simulink model "TRN_V3"  (R2022a)
settings: Solver=FixedStepAuto  StartTime=0.0  StopTime=300  FixedStep=0.04  RelTol=1e-3
PreLoadFcn:
  | load('BusStructureTRNsensor.mat')
InitFcn:
  | %load TRNDataBusPILS.mat
  | %addpath(genpath(cd))
  | 
  | % Add DataBus Path
  | addpath(',,/');
  | addpath('../MAP/');
  | addpath('../MAP/MAP_DB');
  | addpath('../MAP/DVOF');
  | addpath(genpath(cd));
  | load('BusStructureTRN.mat');
  | load('BusStructureDatapump.mat');
undefined symbols (not defined in the file or in its folder): Altitude_INS, INSDataNotValid, Latitude_INS, Longitude_INS, RALTValid, TRN, TRNlib
libraries: simulink_extras x38, aerolibconvert2 x20, dspstat3 x3, sharedtransform x2
(part 2 of 3)

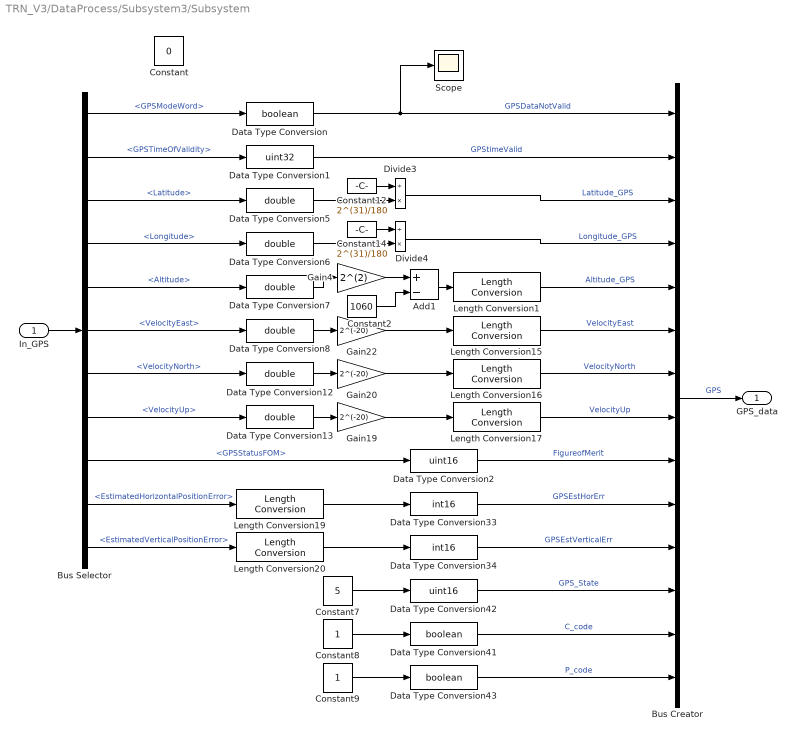
== system TRN_V3/DataProcess/Subsystem3/Subsystem ==
  In_GPS : Inport
  Add1 : Sum  Inputs=+-
  Bus Creator : BusCreator  Inputs=14  OutDataTypeStr=Bus: TRN_GPS
  Bus Selector : BusSelector  OutputSignals=GPSModeWord,GPSTimeOfValidity,Latitude,Longitude,Altitude,VelocityEast,VelocityNorth,VelocityUp,GPSStatusFOM,EstimatedHorizontalPositionError,EstimatedVerticalPositionError
  Constant : Constant  Value=0
  Constant12 : Constant  Value=2^(31)/180
  Constant14 : Constant  Value=2^(31)/180
  Constant2 : Constant  Value=1060
  Constant7 : Constant  Value=5
  Constant8 : Constant
  Constant9 : Constant
  Data Type Conversion : DataTypeConversion  OutDataTypeStr=boolean  SaturateOnIntegerOverflow=off  RndMeth=Floor
  Data Type Conversion1 : DataTypeConversion  OutDataTypeStr=uint32  SaturateOnIntegerOverflow=off  RndMeth=Floor
  Data Type Conversion{5..8,12..13} (6 alike) : DataTypeConversion  OutDataTypeStr=double  SaturateOnIntegerOverflow=off  RndMeth=Floor
  Data Type Conversion2 : DataTypeConversion  OutDataTypeStr=uint16  SaturateOnIntegerOverflow=off  RndMeth=Floor
  Data Type Conversion33 : DataTypeConversion  OutDataTypeStr=int16  SaturateOnIntegerOverflow=off  RndMeth=Floor
  Data Type Conversion34 : DataTypeConversion  OutDataTypeStr=int16  SaturateOnIntegerOverflow=off  RndMeth=Floor
  Data Type Conversion41 : DataTypeConversion  OutDataTypeStr=boolean  SaturateOnIntegerOverflow=off  RndMeth=Floor
  Data Type Conversion42 : DataTypeConversion  OutDataTypeStr=uint16  SaturateOnIntegerOverflow=off  RndMeth=Floor
  Data Type Conversion43 : DataTypeConversion  OutDataTypeStr=boolean  SaturateOnIntegerOverflow=off  RndMeth=Floor
  Divide3 : Product  Inputs=/*
  Divide4 : Product  Inputs=/*
  Gain19 : Gain  Gain=2^(-20)
  Gain20 : Gain  Gain=2^(-20)
  Gain22 : Gain  Gain=2^(-20)
  Gain4 : Gain  Gain=2^(2)
  Length Conversion{1,15..17,19..20} (6 alike) : aerolibconvert2/Length Conversion  IU=ft  OU=m
  Scope : Scope
  GPS_data : Outport
  wires:
  Length Conversion1/1 -> Bus Creator/5  "Altitude_GPS"
  Bus Selector/7 -> Data Type Conversion12/1  "<VelocityNorth>"
  Bus Selector/2 -> Data Type Conversion1/1  "<GPSTimeOfValidity>"
  Bus Selector/3 -> Data Type Conversion5/1  "<Latitude>"
  Gain4/1 -> Add1/1
  Data Type Conversion33/1 -> Bus Creator/10  "GPSEstHorErr"
  Bus Selector/5 -> Data Type Conversion7/1  "<Altitude>"
  Data Type Conversion8/1 -> Gain22/1
  Data Type Conversion41/1 -> Bus Creator/13  "C_code"
  Bus Selector/11 -> Length Conversion20/1  "<EstimatedVerticalPositionError>"
  Gain20/1 -> Length Conversion16/1
  Bus Selector/10 -> Length Conversion19/1  "<EstimatedHorizontalPositionError>"
  Divide3/1 -> Bus Creator/3  "Latitude_GPS"
  Bus Selector/6 -> Data Type Conversion8/1  "<VelocityEast>"
  Data Type Conversion13/1 -> Gain19/1
  Data Type Conversion6/1 -> Divide4/2
  Data Type Conversion34/1 -> Bus Creator/11  "GPSEstVerticalErr"
  Data Type Conversion42/1 -> Bus Creator/12  "GPS_State"
  Gain22/1 -> Length Conversion15/1
  Length Conversion20/1 -> Data Type Conversion34/1
  Data Type Conversion5/1 -> Divide3/2
  Add1/1 -> Length Conversion1/1
  Data Type Conversion1/1 -> Bus Creator/2  "GPStimeValid"
  Gain19/1 -> Length Conversion17/1
  Constant8/1 -> Data Type Conversion41/1
  Data Type Conversion2/1 -> Bus Creator/9  "FigureofMerit"
  Data Type Conversion7/1 -> Gain4/1
  Bus Selector/8 -> Data Type Conversion13/1  "<VelocityUp>"
  Constant7/1 -> Data Type Conversion42/1
  Bus Selector/4 -> Data Type Conversion6/1  "<Longitude>"
  Bus Selector/9 -> Data Type Conversion2/1  "<GPSStatusFOM>"
  Length Conversion17/1 -> Bus Creator/8  "VelocityUp"
  Length Conversion16/1 -> Bus Creator/7  "VelocityNorth"
  Bus Creator/1 -> GPS_data/1  "GPS"
  Data Type Conversion12/1 -> Gain20/1
  Constant2/1 -> Add1/2
  Length Conversion15/1 -> Bus Creator/6  "VelocityEast"
  Length Conversion19/1 -> Data Type Conversion33/1
  Divide4/1 -> Bus Creator/4  "Longitude_GPS"
  Constant9/1 -> Data Type Conversion43/1
  In_GPS/1 -> Bus Selector/1
  Constant14/1 -> Divide4/1
  Constant12/1 -> Divide3/1
  Data Type Conversion43/1 -> Bus Creator/14  "P_code"
  Data Type Conversion/1 -> Scope/1, Bus Creator/1  "GPSDataNotValid"
  Bus Selector/1 -> Data Type Conversion/1  "<GPSModeWord>"

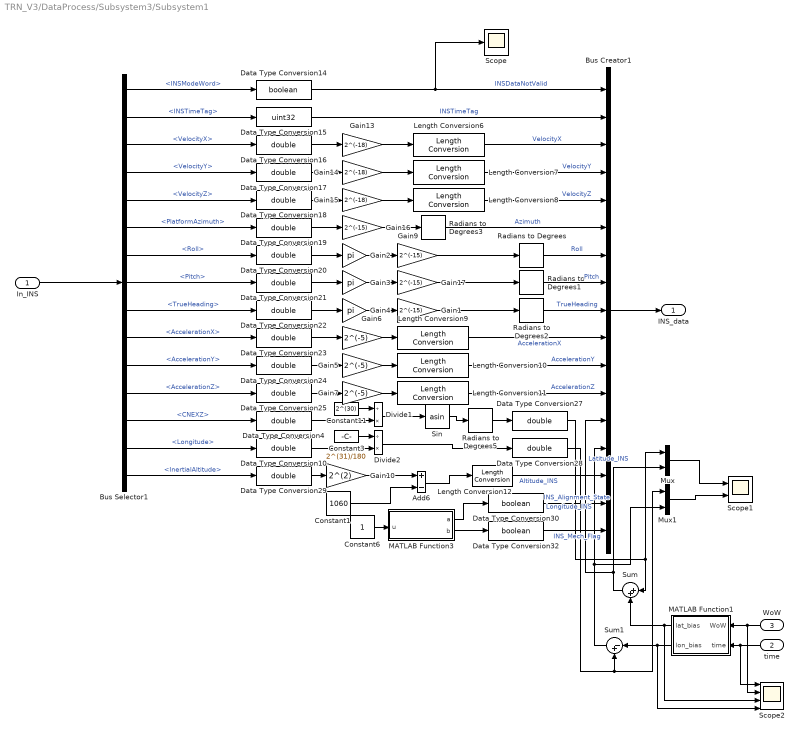
== system TRN_V3/DataProcess/Subsystem3/Subsystem1 ==
  In_INS : Inport
  time : Inport  Port=2
  WoW : Inport  Port=3
  Add6 : Sum  Inputs=+-
  Bus Creator1 : BusCreator  Inputs=17  OutDataTypeStr=Bus: TRN_INS
  Bus Selector1 : BusSelector  OutputSignals=INSModeWord,INSTimeTag,VelocityX,VelocityY,VelocityZ,PlatformAzimuth,Roll,Pitch,TrueHeading,AccelerationX,AccelerationY,AccelerationZ,CNEXZ,Longitude,InertialAltitude
  Constant1 : Constant  Value=1060
  Constant11 : Constant  Value=2^(30)
  Constant3 : Constant  Value=2^(31)/180
  Constant6 : Constant
  Data Type Conversion{4,10,16..25,27..29} (15 alike) : DataTypeConversion  OutDataTypeStr=double  SaturateOnIntegerOverflow=off  RndMeth=Floor
  Data Type Conversion14 : DataTypeConversion  OutDataTypeStr=boolean  SaturateOnIntegerOverflow=off  RndMeth=Floor
  Data Type Conversion15 : DataTypeConversion  OutDataTypeStr=uint32  SaturateOnIntegerOverflow=off  RndMeth=Floor
  Data Type Conversion30 : DataTypeConversion  OutDataTypeStr=boolean  SaturateOnIntegerOverflow=off  RndMeth=Floor
  Data Type Conversion32 : DataTypeConversion  OutDataTypeStr=boolean  SaturateOnIntegerOverflow=off  RndMeth=Floor
  Divide1 : Product  Inputs=/*
  Divide2 : Product  Inputs=/*
  Gain{1,9,16..17} (4 alike) : Gain  Gain=2^(-15)
  Gain10 : Gain  Gain=2^(2)
  Gain13 : Gain  Gain=2^(-18)
  Gain14 : Gain  Gain=2^(-18)
  Gain15 : Gain  Gain=2^(-18)
  Gain2 : Gain  Gain=pi
  Gain3 : Gain  Gain=pi
  Gain4 : Gain  Gain=pi
  Gain5 : Gain  Gain=2^(-5)
  Gain6 : Gain  Gain=2^(-5)
  Gain7 : Gain  Gain=2^(-5)
  Length Conversion{6..12} (7 alike) : aerolibconvert2/Length Conversion  IU=ft  OU=m
  MATLAB Function1 : MATLAB Function  TreatAsAtomicUnit=on
  MATLAB Function3 : MATLAB Function  TreatAsAtomicUnit=on
  Mux : Mux  Inputs=2
  Mux1 : Mux  Inputs=2
  Radians to Degrees{,1..3,5} (5 alike) : simulink_extras/Transformations/Radians to Degrees
  Scope : Scope
  Scope1 : Scope  NumInputPorts=2
  Scope2 : Scope  NumInputPorts=4
  Sin : Trigonometry  Operator=asin
  Sum : Sum  Inputs=|++
  Sum1 : Sum  Inputs=|-+
  INS_data : Outport
  wires:
  Length Conversion6/1 -> Bus Creator1/3  "VelocityX"
  Constant6/1 -> MATLAB Function3/1(u)
  MATLAB Function3/2(b) -> Data Type Conversion32/1
  Data Type Conversion32/1 -> Bus Creator1/17  "INS_Mech_Flag"
  Data Type Conversion22/1 -> Gain4/1
  Length Conversion9/1 -> Bus Creator1/10  "AccelerationX"
  Data Type Conversion29/1 -> Gain10/1
  Radians to Degrees2/1 -> Bus Creator1/9  "TrueHeading"
  Data Type Conversion16/1 -> Gain13/1
  Data Type Conversion18/1 -> Gain15/1
  Data Type Conversion15/1 -> Bus Creator1/2  "INSTimeTag"
  Bus Selector1/14 -> Data Type Conversion10/1  "<Longitude>"
  Radians to Degrees5/1 -> Data Type Conversion27/1
  Data Type Conversion24/1 -> Gain5/1
  Sin/1 -> Radians to Degrees5/1
  Constant1/1 -> Add6/2
  Gain14/1 -> Length Conversion7/1
  Data Type Conversion14/1 -> Scope/1, Bus Creator1/1  "INSDataNotValid"
  Bus Selector1/5 -> Data Type Conversion18/1  "<VelocityZ>"
  Data Type Conversion25/1 -> Gain7/1
  Divide2/1 -> Data Type Conversion28/1
  MATLAB Function3/1(a) -> Data Type Conversion30/1
  Data Type Conversion19/1 -> Gain16/1
  Bus Selector1/10 -> Data Type Conversion23/1  "<AccelerationX>"
  Data Type Conversion20/1 -> Gain2/1
  Bus Selector1/6 -> Data Type Conversion19/1  "<PlatformAzimuth>"
  Data Type Conversion23/1 -> Gain6/1
  Bus Selector1/7 -> Data Type Conversion20/1  "<Roll>"
  Bus Selector1/2 -> Data Type Conversion15/1  "<INSTimeTag>"
  Bus Selector1/4 -> Data Type Conversion17/1  "<VelocityY>"
  Bus Selector1/3 -> Data Type Conversion16/1  "<VelocityX>"
  Add6/1 -> Length Conversion12/1
  Bus Selector1/15 -> Data Type Conversion29/1  "<InertialAltitude>"
  Bus Selector1/12 -> Data Type Conversion25/1  "<AccelerationZ>"
  Bus Selector1/13 -> Data Type Conversion4/1  "<CNEXZ>"
  Data Type Conversion4/1 -> Divide1/2
  Bus Selector1/9 -> Data Type Conversion22/1  "<TrueHeading>"
  Gain15/1 -> Length Conversion8/1
  Bus Selector1/11 -> Data Type Conversion24/1  "<AccelerationY>"
  Length Conversion12/1 -> Bus Creator1/15  "Altitude_INS"
  Gain6/1 -> Length Conversion9/1
  Data Type Conversion21/1 -> Gain3/1
  Length Conversion8/1 -> Bus Creator1/5  "VelocityZ"
  Data Type Conversion17/1 -> Gain14/1
  Radians to Degrees1/1 -> Bus Creator1/8  "Pitch"
  Length Conversion7/1 -> Bus Creator1/4  "VelocityY"
  Constant3/1 -> Divide2/1
  Gain5/1 -> Length Conversion10/1
  Length Conversion10/1 -> Bus Creator1/11  "AccelerationY"
  Gain7/1 -> Length Conversion11/1
  Radians to Degrees/1 -> Bus Creator1/7  "Roll"
  Divide1/1 -> Sin/1
  Bus Selector1/8 -> Data Type Conversion21/1  "<Pitch>"
  Data Type Conversion10/1 -> Divide2/2
  Data Type Conversion30/1 -> Bus Creator1/16  "INS_Alignment_State"
  Gain10/1 -> Add6/1
  Radians to Degrees3/1 -> Bus Creator1/6  "Azimuth"
  Length Conversion11/1 -> Bus Creator1/12  "AccelerationZ"
  Constant11/1 -> Divide1/1
  Gain16/1 -> Radians to Degrees3/1
  Gain13/1 -> Length Conversion6/1
  Bus Creator1/1 -> INS_data/1
  In_INS/1 -> Bus Selector1/1
  Gain3/1 -> Gain17/1
  Gain4/1 -> Gain1/1
  Gain2/1 -> Gain9/1
  Gain9/1 -> Radians to Degrees/1
  Gain17/1 -> Radians to Degrees1/1
  Gain1/1 -> Radians to Degrees2/1
  Bus Selector1/1 -> Data Type Conversion14/1  "<INSModeWord>"
  Sum/1 -> Bus Creator1/13, Mux/2  "Latitude_INS"
  MATLAB Function1/1(lat_bias) -> Scope2/3, Sum/2
  Sum1/1 -> Mux1/2, Bus Creator1/14  "Longitude_INS"
  MATLAB Function1/2(lon_bias) -> Scope2/4, Sum1/1
  Mux/1 -> Scope1/1
  Mux1/1 -> Scope1/2
  Data Type Conversion27/1 -> Sum/1, Mux/1
  Data Type Conversion28/1 -> Sum1/2, Mux1/1
  WoW/1 -> Scope2/2, MATLAB Function1/1(WoW)
  time/1 -> Scope2/1, MATLAB Function1/2(time)

== system TRN_V3/DataProcess/Subsystem3/Subsystem4 ==
  In_RALT : Inport
  Add5 : Sum  Inputs=+-
  Bus Creator2 : BusCreator  Inputs=3  OutDataTypeStr=Bus: TRN_RALT
  Bus Selector2 : BusSelector  OutputSignals=RALTModeWord,TimeTag,RadarAltitude
  Constant4 : Constant  Value=50
  Constant5 : Constant  Value=0.625
  Data Type Conversion3 : DataTypeConversion  OutDataTypeStr=double  SaturateOnIntegerOverflow=off  RndMeth=Floor
  Data Type Conversion31 : DataTypeConversion  OutDataTypeStr=uint32  SaturateOnIntegerOverflow=off  RndMeth=Floor
  Data Type Conversion35 : DataTypeConversion  OutDataTypeStr=boolean  SaturateOnIntegerOverflow=off  RndMeth=Floor
  Length Conversion2 : aerolibconvert2/Length Conversion  IU=ft  OU=m
  Product1 : Product
  RALT_data : Outport
  wires:
  Length Conversion2/1 -> Bus Creator2/3  "RALTAltitude"
  Constant4/1 -> Add5/2
  Bus Creator2/1 -> RALT_data/1  "RALT"
  In_RALT/1 -> Bus Selector2/1
  Data Type Conversion35/1 -> Bus Creator2/1  "RALTValid"
  Add5/1 -> Length Conversion2/1
  Bus Selector2/3 -> Data Type Conversion3/1  "<RadarAltitude>"
  Data Type Conversion3/1 -> Product1/1
  Product1/1 -> Add5/1
  Constant5/1 -> Product1/2
  Data Type Conversion31/1 -> Bus Creator2/2  "RALTTimeTag"
  Bus Selector2/2 -> Data Type Conversion31/1  "<TimeTag>"
  Bus Selector2/1 -> Data Type Conversion35/1  "<RALTModeWord>"

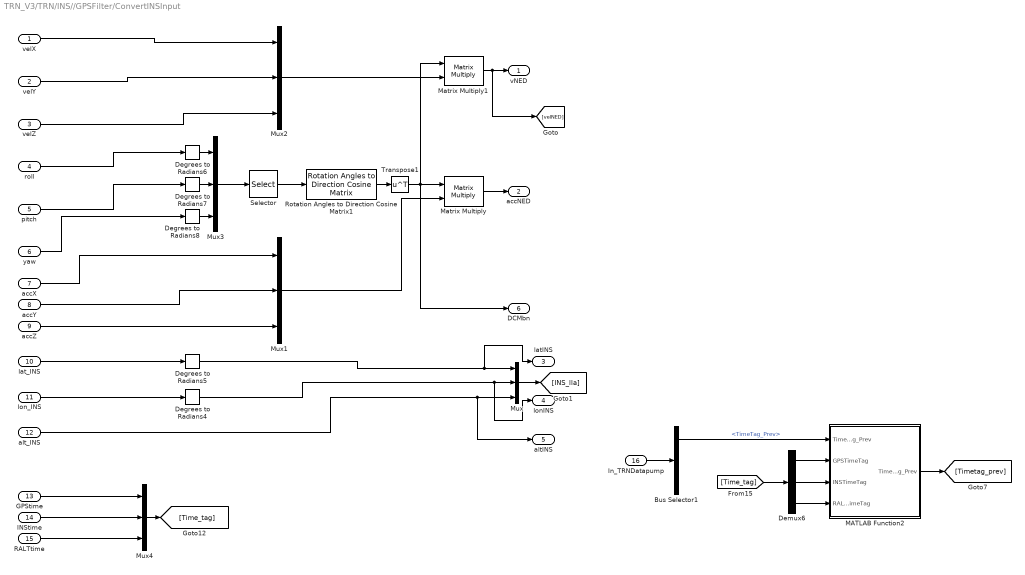
== system TRN_V3/TRN/INS//GPSFilter/ConvertINSInput ==
  velX : Inport
  velY : Inport  Port=2
  velZ : Inport  Port=3
  roll : Inport  Port=4
  pitch : Inport  Port=5
  yaw : Inport  Port=6
  accX : Inport  Port=7
  accY : Inport  Port=8
  accZ : Inport  Port=9
  lat_INS : Inport  Port=10
  lon_INS : Inport  Port=11
  alt_INS : Inport  Port=12
  GPStime : Inport  Port=13
  INStime : Inport  Port=14
  RALTtime : Inport  Port=15
  In_TRNDatapump : Inport  Port=16  OutDataTypeStr=Bus: TRNDatapump  PortDimensions=1
  Bus Selector1 : BusSelector  OutputSignals=TimeTag_Prev,Result_Prev,xu
  Degrees to Radians{4..8} (5 alike) : simulink_extras/Transformations/Degrees to Radians
  Demux6 : Demux  Outputs=3
  MATLAB Function2 : MATLAB Function  TreatAsAtomicUnit=on
  Matrix Multiply : Product  Multiplication=Matrix(*)
  Matrix Multiply1 : Product  Multiplication=Matrix(*)
  Mux{,1..4} (5 alike) : Mux  Inputs=3
  Rotation Angles to Direction Cosine Matrix1 : sharedtransform/Rotation Angles to Direction Cosine Matrix  rotationOrder=ZYX  aMode=aMode
      settings: SourceProductBaseCode=AE
  Selector : Selector  InputPortWidth=3  IndexOptions=Index vector (dialog)  Indices=[3 2 1]  OutputSizes=1
  Transpose1 : Math  Operator=transpose  SignedPower=on
  vNED : Outport  VectorParamsAs1DForOutWhenUnconnected=off
  accNED : Outport  Port=2  VectorParamsAs1DForOutWhenUnconnected=off
  latINS : Outport  Port=3  VectorParamsAs1DForOutWhenUnconnected=off
  lonINS : Outport  Port=4  VectorParamsAs1DForOutWhenUnconnected=off
  altINS : Outport  Port=5  VectorParamsAs1DForOutWhenUnconnected=off
  DCMbn : Outport  Port=6  VectorParamsAs1DForOutWhenUnconnected=off
  wires:
  Degrees to Radians6/1 -> Mux3/1
  Degrees to Radians7/1 -> Mux3/2
  Selector/1 -> Rotation Angles to Direction Cosine Matrix1/1
  Transpose1/1 -> DCMbn/1, Matrix Multiply/1, Matrix Multiply1/1
  Rotation Angles to Direction Cosine Matrix1/1 -> Transpose1/1
  Mux1/1 -> Matrix Multiply/2
  Mux3/1 -> Selector/1
  Matrix Multiply1/1 -> [velNED], vNED/1
  Degrees to Radians8/1 -> Mux3/3
  Matrix Multiply/1 -> accNED/1
  Mux2/1 -> Matrix Multiply1/2
  alt_INS/1 -> altINS/1, Mux/3
  lon_INS/1 -> Degrees to Radians4/1
  accZ/1 -> Mux1/3
  accY/1 -> Mux1/2
  yaw/1 -> Degrees to Radians8/1
  velX/1 -> Mux2/1
  velZ/1 -> Mux2/3
  velY/1 -> Mux2/2
  accX/1 -> Mux1/1
  Degrees to Radians5/1 -> latINS/1, Mux/1
  Degrees to Radians4/1 -> lonINS/1, Mux/2
  pitch/1 -> Degrees to Radians7/1
  lat_INS/1 -> Degrees to Radians5/1
  roll/1 -> Degrees to Radians6/1
  Mux/1 -> [INS_lla]
  Demux6/2 -> MATLAB Function2/3(INSTimeTag)
  In_TRNDatapump/1 -> Bus Selector1/1
  RALTtime/1 -> Mux4/3
  Demux6/3 -> MATLAB Function2/4(RALTTimeTag)
  [Time_tag] -> Demux6/1
  GPStime/1 -> Mux4/1
  Bus Selector1/1 -> MATLAB Function2/1("TimeTag_Prev ")  "<TimeTag_Prev>"
  MATLAB Function2/1(TimeTag_Prev) -> [Timetag_prev]
  INStime/1 -> Mux4/2
  Mux4/1 -> [Time_tag]
  Demux6/1 -> MATLAB Function2/2(GPSTimeTag)

== system TRN_V3/TRN/TRNSchedulerDTNS1/AcquisitionCSU/AcquisitionCSU ==
  In_TRNInput : Inport  OutDataTypeStr=Bus: TRNInput
  In_TRNDatapump : Inport  Port=2  OutDataTypeStr=Bus: TRNDatapump
  Bus Selector1 : BusSelector  OutputSignals=profileCnt
  ConvertTRNInput : Subsystem  TreatAsAtomicUnit=on
  CorrelationAnalysis function : MATLAB Function  TreatAsAtomicUnit=on
  Data Store Read : DataStoreRead  DataStoreName=BatchProf  IndexOptions=Index vector (dialog)  Indices=1  OutputSizes=1
  Data Store Write : DataStoreWrite  DataStoreName=BatchProf  IndexOptions=Index vector (dialog)  Indices=1  OutputSizes=1
  Radians to Degrees : simulink_extras/Transformations/Radians to Degrees
  Radians to Degrees1 : simulink_extras/Transformations/Radians to Degrees
  Resolution : Constant  Value=3 * 0.000277777777777777 * 0.0174532925199433
  Scope : Scope  NumInputPorts=4
  Scope1 : Scope
  StoreProfile function : MATLAB Function  TreatAsAtomicUnit=on
  MAD : Outport  VectorParamsAs1DForOutWhenUnconnected=off
  profileCnt : Outport  Port=2  VectorParamsAs1DForOutWhenUnconnected=off
  posUpdate : Outport  Port=3  VectorParamsAs1DForOutWhenUnconnected=off
  residual : Outport  Port=4  VectorParamsAs1DForOutWhenUnconnected=off
  wires:
  ConvertTRNInput/9(flagINS) -> StoreProfile function/11(flagINS)
  CorrelationAnalysis function/8(sum) -> Scope/4
  CorrelationAnalysis function/7(hDEM) -> Scope/3
  CorrelationAnalysis function/5(lonTemp) -> Radians to Degrees1/1
  CorrelationAnalysis function/6(latTemp) -> Radians to Degrees/1
  In_TRNDatapump/1 -> Bus Selector1/1
  In_TRNInput/1 -> ConvertTRNInput/1(TRNInput)
  Bus Selector1/1 -> StoreProfile function/2("profileCnt ")  "<profileCnt>"
  ConvertTRNInput/1(latINS) -> StoreProfile function/3(latINS)
  ConvertTRNInput/2(lonINS) -> StoreProfile function/4(lonINS)
  ConvertTRNInput/3(altINS) -> StoreProfile function/5(altINS)
  ConvertTRNInput/4(altRALT) -> Scope1/1, StoreProfile function/6(RALT)
  Resolution/1 -> CorrelationAnalysis function/3(resolution)
  StoreProfile function/1(batchProfile) -> CorrelationAnalysis function/1("batchProfile ")
  StoreProfile function/2(profileCnt) -> CorrelationAnalysis function/2(profileCnt), profileCnt/1
  CorrelationAnalysis function/2(MAD) -> MAD/1
  CorrelationAnalysis function/1(posUpdate) -> posUpdate/1
  CorrelationAnalysis function/3(residual) -> residual/1
  StoreProfile function/3(gridSize) -> CorrelationAnalysis function/4(gridSize)
  Data Store Read/1 -> StoreProfile function/1("batchProfile ")
  CorrelationAnalysis function/4(batchProfile) -> Data Store Write/1
  ConvertTRNInput/5(latGPS) -> StoreProfile function/7(latGPS)
  ConvertTRNInput/6(lonGPS) -> StoreProfile function/8(lonGPS)
  ConvertTRNInput/7(altGPS) -> StoreProfile function/9(altGPS)
  ConvertTRNInput/8(flagGPS) -> StoreProfile function/10(flagGPS)
  Radians to Degrees/1 -> Scope/1
  Radians to Degrees1/1 -> Scope/2

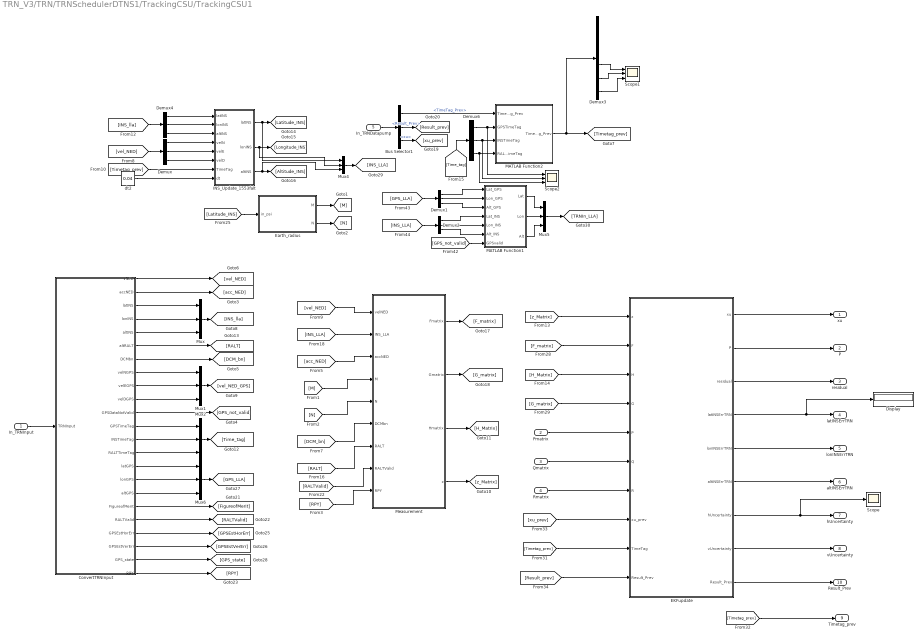
== system TRN_V3/TRN/TRNSchedulerDTNS1/TrackingCSU/TrackingCSU1 ==
  In_TRNInput : Inport  OutDataTypeStr=Bus: TRNInput
  Pmatrix : Inport  Port=2
  Qmatrix : Inport  Port=3
  Rmatrix : Inport  Port=4
  In_TRNDatapump : Inport  Port=5  OutDataTypeStr=Bus: TRNDatapump  PortDimensions=1
  Bus Selector1 : BusSelector  OutputSignals=TimeTag_Prev,Result_Prev,xu
  ConvertTRNInput : Subsystem  TreatAsAtomicUnit=on
  Demux{,1..2,4,6} (5 alike) : Demux  Outputs=3
  Demux3 : Demux  Outputs=6
  Display : Display
  EKFupdate : Subsystem
  Earth_radius : MATLAB Function  TreatAsAtomicUnit=on
  INS_Update_1553falt : MATLAB Function  TreatAsAtomicUnit=on
  MATLAB Function1 : MATLAB Function  TreatAsAtomicUnit=on
  MATLAB Function2 : MATLAB Function  TreatAsAtomicUnit=on
  Measurement : Subsystem
  Mux{,1..2,4..6} (6 alike) : Mux  Inputs=3
  Scope : Scope
  Scope1 : Scope  NumInputPorts=3
  Scope2 : Scope  NumInputPorts=3
  dt2 : Constant  Value=0.04  OutDataTypeStr=double
  xu : Outport
  P : Outport  Port=2
  residual : Outport  Port=3
  latINSErrTRN : Outport  Port=4
  lonINSErrTRN : Outport  Port=5
  altINSErrTRN : Outport  Port=6
  hUncertainty : Outport  Port=7
  vUncertainty : Outport  Port=8
  Timetag_prev : Outport  Port=9
  Result_Prev : Outport  Port=10
  wires:
  Mux5/1 -> [TRNIn_LLA]
  MATLAB Function1/3(Alt) -> Mux5/3
  MATLAB Function1/1(Lat) -> Mux5/1
  MATLAB Function1/2(Lon) -> Mux5/2
  Demux2/3 -> MATLAB Function1/6(Alt_INS)
  Demux2/2 -> MATLAB Function1/5(Lon_INS)
  Demux2/1 -> MATLAB Function1/4(Lat_INS)
  [INS_LLA] -> Demux2/1
  Mux4/1 -> [INS_LLA]
  Demux1/3 -> MATLAB Function1/3(Alt_GPS)
  Demux1/1 -> MATLAB Function1/1(Lat_GPS)
  Demux1/2 -> MATLAB Function1/2(Lon_GPS)
  [GPS_LLA] -> Demux1/1
  [GPS_not_valid] -> MATLAB Function1/7(GPSvalid)
  ConvertTRNInput/22(GPS_state) -> [GPS_state]
  ConvertTRNInput/21(GPSEstVerErr) -> [GPSEstVerErr]
  ConvertTRNInput/20(GPSEstHorErr) -> [GPSEstHorErr]
  Demux/3 -> INS_Update_1553falt/6(velD)
  Demux/1 -> INS_Update_1553falt/4(velN)
  Demux/2 -> INS_Update_1553falt/5(velE)
  dt2/1 -> INS_Update_1553falt/8(dt)
  Bus Selector1/1 -> MATLAB Function2/1("TimeTag_Prev ")  "<TimeTag_Prev>"
  In_TRNDatapump/1 -> Bus Selector1/1
  INS_Update_1553falt/3(altINS) -> [Altitude_INS], Mux4/3
  In_TRNInput/1 -> ConvertTRNInput/1(TRNInput)
  INS_Update_1553falt/1(latINS) -> [Latitude_INS], Mux4/1
  INS_Update_1553falt/2(lonINS) -> [Longitude_INS], Mux4/2
  ConvertTRNInput/2(accNED) -> [acc_NED]
  ConvertTRNInput/11(GPSDataNotValid) -> [GPS_not_valid]
  ConvertTRNInput/7(DCMbn) -> [DCM_bn]
  ConvertTRNInput/1(vNED) -> [vel_NED]
  [vel_NED] -> Demux/1
  [Timetag_prev] -> INS_Update_1553falt/7(TimeTag)
  ConvertTRNInput/3(latINS) -> Mux/1
  ConvertTRNInput/4(lonINS) -> Mux/2
  ConvertTRNInput/5(altINS) -> Mux/3
  Mux/1 -> [INS_lla]
  [INS_lla] -> Demux4/1
  Demux4/2 -> INS_Update_1553falt/2("lonINS ")
  Demux4/1 -> INS_Update_1553falt/1("latINS ")
  Demux4/3 -> INS_Update_1553falt/3("altINS ")
  ConvertTRNInput/10(velDGPS) -> Mux1/3
  ConvertTRNInput/9(velEGPS) -> Mux1/2
  Mux1/1 -> [vel_NED_GPS]
  ConvertTRNInput/8(velNGPS) -> Mux1/1
  Mux2/1 -> [Time_tag]
  ConvertTRNInput/12(GPSTimeTag) -> Mux2/1
  ConvertTRNInput/13(INSTimeTag) -> Mux2/2
  ConvertTRNInput/14(RALTTimeTag) -> Mux2/3
  [Time_tag] -> Demux6/1
  Demux6/1 -> Scope2/1, MATLAB Function2/2(GPSTimeTag)
  Demux6/2 -> Scope2/2, MATLAB Function2/3(INSTimeTag)
  Demux6/3 -> Scope2/3, MATLAB Function2/4(RALTTimeTag)
  ConvertTRNInput/6(altRALT) -> [RALT]
  [Timetag_prev] -> Timetag_prev/1
  Bus Selector1/3 -> [xu_prev]  "<xu>"
  Bus Selector1/2 -> [Result_prev]  "<Result_Prev>"
  Measurement/1(Fmatrix) -> [F_matrix]
  Measurement/2(Gmatrix) -> [G_matrix]
  Measurement/3(Hmatrix) -> [H_Matrix]
  Measurement/4(z) -> [z_Matrix]
  [z_Matrix] -> EKFupdate/1(z)
  [F_matrix] -> EKFupdate/2(F)
  [H_Matrix] -> EKFupdate/3(H)
  [G_matrix] -> EKFupdate/4(G)
  Pmatrix/1 -> EKFupdate/5("P ")
  Qmatrix/1 -> EKFupdate/6(Q)
  Rmatrix/1 -> EKFupdate/7(R)
  [xu_prev] -> EKFupdate/8(xu_prev)
  [Timetag_prev] -> EKFupdate/9(TimeTag)
  [Result_prev] -> EKFupdate/10("Result_Prev ")
  EKFupdate/1(xu) -> xu/1
  EKFupdate/2(P) -> P/1
  EKFupdate/3(residual) -> residual/1
  EKFupdate/8(vUncertainty) -> vUncertainty/1
  EKFupdate/4(latINSErrTRN) -> Display/1, latINSErrTRN/1
  EKFupdate/5(lonINSErrTRN) -> lonINSErrTRN/1
  EKFupdate/6(altINSErrTRN) -> altINSErrTRN/1
  EKFupdate/9(Result_Prev) -> Result_Prev/1
  ConvertTRNInput/18(FigureofMerit) -> [FigureofMerit]
  EKFupdate/7(hUncertainty) -> Scope/1, hUncertainty/1
  ConvertTRNInput/19(RALTValid) -> [RALTValid]
  [RALTValid] -> Measurement/8(RALTValid)
  [vel_NED] -> Measurement/1(velNED)
  [INS_LLA] -> Measurement/2(INS_LLA)
  [acc_NED] -> Measurement/3(accNED)
  [M] -> Measurement/4(M)
  [N] -> Measurement/5(N)
  [Latitude_INS] -> Earth_radius/1(in_psi)
  Earth_radius/1(M) -> [M]
  Earth_radius/2(N) -> [N]
  ConvertTRNInput/15(latGPS) -> Mux6/1
  ConvertTRNInput/16(lonGPS) -> Mux6/2
  ConvertTRNInput/17(altGPS) -> Mux6/3
  Mux6/1 -> [GPS_LLA]
  [RALT] -> Measurement/7(RALT)
  [DCM_bn] -> Measurement/6(DCMbn)
  ConvertTRNInput/23(RPY) -> [RPY]
  [RPY] -> Measurement/9(RPY)
  MATLAB Function2/1(TimeTag_Prev) -> Demux3/1, [Timetag_prev]
  Demux3/4 -> Scope1/1
  Demux3/5 -> Scope1/2
  Demux3/6 -> Scope1/3

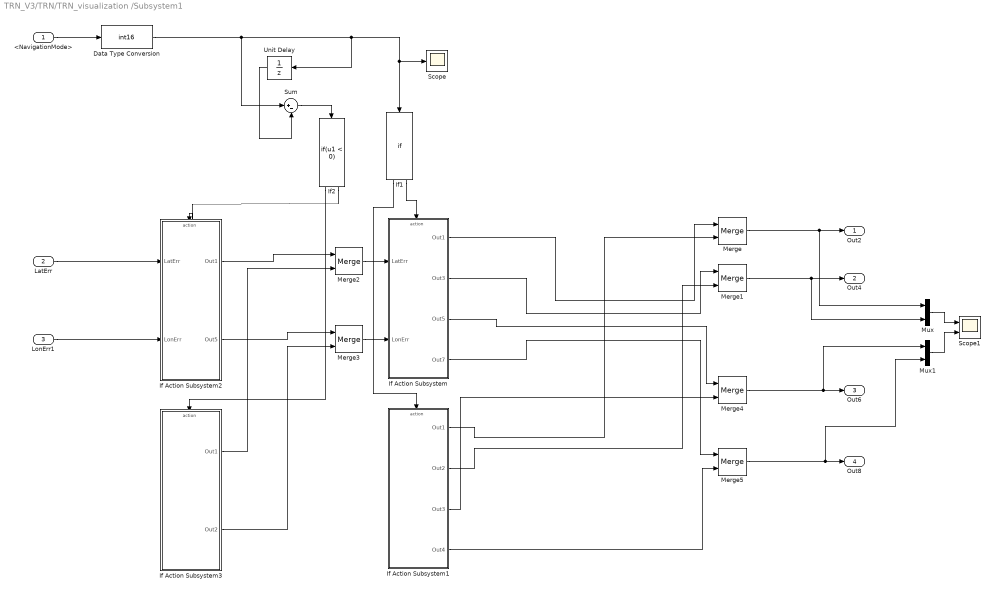
== system TRN_V3/TRN/TRN_visualization /Subsystem1 ==
  <NavigationMode> : Inport
  LatErr : Inport  Port=2
  LonErr1 : Inport  Port=3
  Data Type Conversion : DataTypeConversion  OutDataTypeStr=int16  SaturateOnIntegerOverflow=off  RndMeth=Floor
  If Action Subsystem : Subsystem  TreatAsAtomicUnit=on
  If Action Subsystem1 : Subsystem  TreatAsAtomicUnit=on
  If Action Subsystem2 : Subsystem  TreatAsAtomicUnit=on
  If Action Subsystem3 : Subsystem  TreatAsAtomicUnit=on
  If1 : If
  If2 : If  IfExpression=u1 < 0
  Merge{,1..5} (6 alike) : Merge
  Mux : Mux  Inputs=2
  Mux1 : Mux  Inputs=2
  Scope : Scope
  Scope1 : Scope  NumInputPorts=2
  Sum : Sum  Inputs=|+-
  Unit Delay : UnitDelay  SampleTime=-1  HasFrameUpgradeWarning=on
  Out2 : Outport
  Out4 : Outport  Port=2
  Out6 : Outport  Port=3
  Out8 : Outport  Port=4
  wires:
  If Action Subsystem3/2(Out2) -> Merge3/2
  If Action Subsystem2/2(Out5) -> Merge3/1
  If Action Subsystem3/1(Out1) -> Merge2/2
  If Action Subsystem2/1(Out1) -> Merge2/1
  Merge3/1 -> If Action Subsystem/2(LonErr)
  Merge2/1 -> If Action Subsystem/1(LatErr)
  LonErr1/1 -> If Action Subsystem2/2(LonErr)
  LatErr/1 -> If Action Subsystem2/1(LatErr)
  If2/1 -> If Action Subsystem3/Action
  If2/2 -> If Action Subsystem2/Action
  Sum/1 -> If2/1
  Unit Delay/1 -> Sum/2
  Mux1/1 -> Scope1/2
  Mux/1 -> Scope1/1
  <NavigationMode>/1 -> Data Type Conversion/1
  If Action Subsystem1/4(Out4) -> Merge5/2
  If Action Subsystem1/3(Out3) -> Merge4/2
  If Action Subsystem/4(Out7) -> Merge5/1
  If Action Subsystem/3(Out5) -> Merge4/1
  If Action Subsystem/2(Out3) -> Merge1/1
  Merge1/1 -> Out4/1, Mux/2
  Merge/1 -> Out2/1, Mux/1
  If1/1 -> If Action Subsystem1/Action
  If Action Subsystem1/1(Out1) -> Merge/2
  If Action Subsystem1/2(Out2) -> Merge1/2
  Data Type Conversion/1 -> Sum/1, Scope/1, If1/1, Unit Delay/1
  Merge4/1 -> Out6/1, Mux1/1
  Merge5/1 -> Out8/1, Mux1/2
  If1/2 -> If Action Subsystem/Action
  If Action Subsystem/1(Out1) -> Merge/1

== system TRN_V3/TRN/TRNSchedulerDTNS1/AcquisitionCSU/AcquisitionCSU/ConvertTRNInput ==
  TRNInput : Inport  OutDataTypeStr=Bus: TRNInput
  Bus Selector1 : BusSelector  OutputSignals=Latitude_INS,Longitude_INS,Altitude_INS,RALTAltitude,GPSDataNotValid,Latitude_GPS,Longitude_GPS,Altitude_GPS,INSDataNotValid
  Degrees to Radians{1..2,4..5} (4 alike) : simulink_extras/Transformations/Degrees to Radians
  latINS : Outport  VectorParamsAs1DForOutWhenUnconnected=off
  lonINS : Outport  Port=2  VectorParamsAs1DForOutWhenUnconnected=off
  altINS : Outport  Port=3  VectorParamsAs1DForOutWhenUnconnected=off
  altRALT : Outport  Port=4  VectorParamsAs1DForOutWhenUnconnected=off
  latGPS : Outport  Port=5  VectorParamsAs1DForOutWhenUnconnected=off
  lonGPS : Outport  Port=6  VectorParamsAs1DForOutWhenUnconnected=off
  altGPS : Outport  Port=7  VectorParamsAs1DForOutWhenUnconnected=off
  flagGPS : Outport  Port=8  VectorParamsAs1DForOutWhenUnconnected=off
  flagINS : Outport  Port=9  VectorParamsAs1DForOutWhenUnconnected=off
  wires:
  Bus Selector1/9 -> flagINS/1  "<INSDataNotValid>"
  Bus Selector1/2 -> Degrees to Radians4/1  "<Longitude_INS>"
  Bus Selector1/1 -> Degrees to Radians5/1  "<Latitude_INS>"
  Bus Selector1/4 -> altRALT/1  "<RALTAltitude>"
  Degrees to Radians4/1 -> lonINS/1
  Degrees to Radians5/1 -> latINS/1
  TRNInput/1 -> Bus Selector1/1
  Bus Selector1/3 -> altINS/1  "<Altitude_INS>"
  Bus Selector1/5 -> flagGPS/1  "<GPSDataNotValid>"
  Bus Selector1/6 -> Degrees to Radians1/1  "<Latitude_GPS>"
  Bus Selector1/7 -> Degrees to Radians2/1  "<Longitude_GPS>"
  Bus Selector1/8 -> altGPS/1  "<Altitude_GPS>"
  Degrees to Radians2/1 -> lonGPS/1
  Degrees to Radians1/1 -> latGPS/1

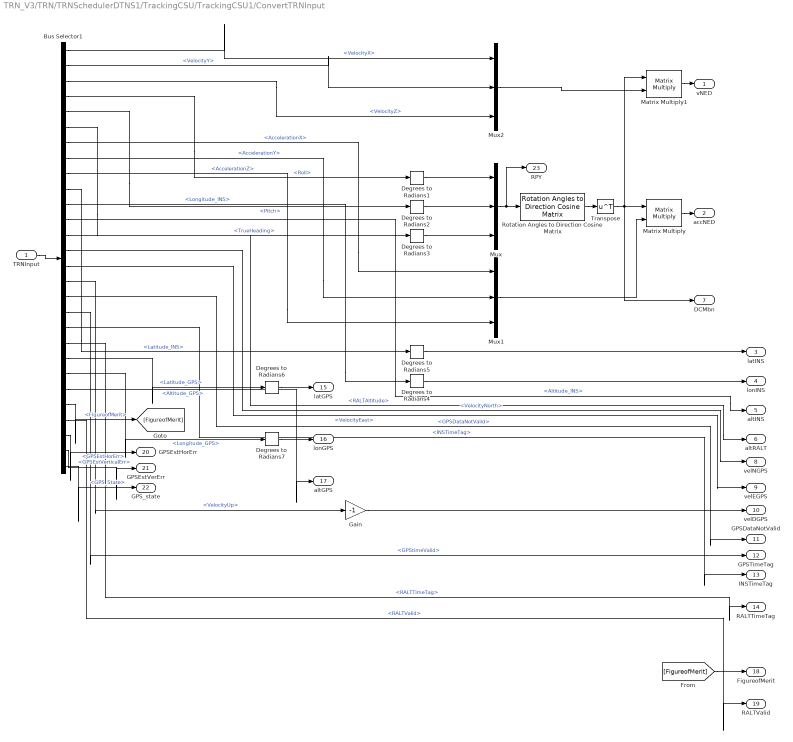
== system TRN_V3/TRN/TRNSchedulerDTNS1/TrackingCSU/TrackingCSU1/ConvertTRNInput ==
  TRNInput : Inport
  Bus Selector1 : BusSelector  OutputSignals=VelocityX,VelocityY,VelocityZ,Roll,Pitch,TrueHeading,AccelerationX,AccelerationY,AccelerationZ,Latitude_INS,Longitude_INS,Altitude_INS,RALTAltitude,VelocityNorth,VelocityEast,VelocityUp,GPSDataNotValid,GPStimeValid,INSTimeTag,RALTTimeTag,Latitude_GPS,Longitude_GPS,Altitude_GPS,FigureofMerit,RALTValid,GPSEstHorErr,GPSEstVerticalErr,GPS_State
  Degrees to Radians{1..7} (7 alike) : simulink_extras/Transformations/Degrees to Radians
  Gain : Gain  Gain=-1
  Matrix Multiply : Product  Multiplication=Matrix(*)
  Matrix Multiply1 : Product  Multiplication=Matrix(*)
  Mux : Mux  Inputs=3
  Mux1 : Mux  Inputs=3
  Mux2 : Mux  Inputs=3
  Rotation Angles to Direction Cosine Matrix : sharedtransform/Rotation Angles to Direction Cosine Matrix  rotationOrder=ZYX  aMode=aMode
      settings: SourceProductBaseCode=AE,PW,DR,MT,VE
  Transpose : Math  Operator=transpose  SignedPower=on
  vNED : Outport  VectorParamsAs1DForOutWhenUnconnected=off
  accNED : Outport  Port=2  VectorParamsAs1DForOutWhenUnconnected=off
  latINS : Outport  Port=3  VectorParamsAs1DForOutWhenUnconnected=off
  lonINS : Outport  Port=4  VectorParamsAs1DForOutWhenUnconnected=off
  altINS : Outport  Port=5  VectorParamsAs1DForOutWhenUnconnected=off
  altRALT : Outport  Port=6  VectorParamsAs1DForOutWhenUnconnected=off
  DCMbn : Outport  Port=7  VectorParamsAs1DForOutWhenUnconnected=off
  velNGPS : Outport  Port=8  VectorParamsAs1DForOutWhenUnconnected=off
  velEGPS : Outport  Port=9  VectorParamsAs1DForOutWhenUnconnected=off
  velDGPS : Outport  Port=10  VectorParamsAs1DForOutWhenUnconnected=off
  GPSDataNotValid : Outport  Port=11  VectorParamsAs1DForOutWhenUnconnected=off
  GPSTimeTag : Outport  Port=12  VectorParamsAs1DForOutWhenUnconnected=off
  INSTimeTag : Outport  Port=13  VectorParamsAs1DForOutWhenUnconnected=off
  RALTTimeTag : Outport  Port=14  VectorParamsAs1DForOutWhenUnconnected=off
  latGPS : Outport  Port=15
  lonGPS : Outport  Port=16
  altGPS : Outport  Port=17
  FigureofMerit : Outport  Port=18
  RALTValid : Outport  Port=19
  GPSEstHorErr : Outport  Port=20
  GPSEstVerErr : Outport  Port=21
  GPS_state : Outport  Port=22
  RPY : Outport  Port=23  VectorParamsAs1DForOutWhenUnconnected=off
  wires:
  Bus Selector1/28 -> GPS_state/1  "<GPS_State>"
  Bus Selector1/27 -> GPSEstVerErr/1  "<GPSEstVerticalErr>"
  Bus Selector1/26 -> GPSEstHorErr/1  "<GPSEstHorErr>"
  Bus Selector1/23 -> altGPS/1  "<Altitude_GPS>"
  Bus Selector1/22 -> Degrees to Radians7/1  "<Longitude_GPS>"
  Degrees to Radians7/1 -> lonGPS/1
  Bus Selector1/20 -> RALTTimeTag/1  "<RALTTimeTag>"
  Bus Selector1/19 -> INSTimeTag/1  "<INSTimeTag>"
  Bus Selector1/18 -> GPSTimeTag/1  "<GPStimeValid>"
  Bus Selector1/17 -> GPSDataNotValid/1  "<GPSDataNotValid>"
  Gain/1 -> velDGPS/1
  Bus Selector1/16 -> Gain/1  "<VelocityUp>"
  Bus Selector1/15 -> velEGPS/1  "<VelocityEast>"
  Bus Selector1/14 -> velNGPS/1  "<VelocityNorth>"
  Bus Selector1/12 -> altINS/1  "<Altitude_INS>"
  Bus Selector1/3 -> Mux2/3  "<VelocityZ>"
  Bus Selector1/1 -> Mux2/1  "<VelocityX>"
  Bus Selector1/4 -> Degrees to Radians1/1  "<Roll>"
  Bus Selector1/2 -> Mux2/2  "<VelocityY>"
  TRNInput/1 -> Bus Selector1/1
  Bus Selector1/6 -> Degrees to Radians3/1  "<TrueHeading>"
  Degrees to Radians2/1 -> Mux/2
  Degrees to Radians3/1 -> Mux/3
  Mux/1 -> RPY/1, Rotation Angles to Direction Cosine Matrix/1
  Bus Selector1/7 -> Mux1/1  "<AccelerationX>"
  Bus Selector1/5 -> Degrees to Radians2/1  "<Pitch>"
  Degrees to Radians1/1 -> Mux/1
  Bus Selector1/9 -> Mux1/3  "<AccelerationZ>"
  Bus Selector1/8 -> Mux1/2  "<AccelerationY>"
  Degrees to Radians5/1 -> latINS/1
  Matrix Multiply1/1 -> vNED/1
  Degrees to Radians4/1 -> lonINS/1
  Matrix Multiply/1 -> accNED/1
  Bus Selector1/13 -> altRALT/1  "<RALTAltitude>"
  Mux1/1 -> Matrix Multiply/2
  Bus Selector1/10 -> Degrees to Radians5/1  "<Latitude_INS>"
  Transpose/1 -> Matrix Multiply1/1, Matrix Multiply/1, DCMbn/1
  Mux2/1 -> Matrix Multiply1/2
  Rotation Angles to Direction Cosine Matrix/1 -> Transpose/1
  Bus Selector1/11 -> Degrees to Radians4/1  "<Longitude_INS>"
  Degrees to Radians6/1 -> latGPS/1
  Bus Selector1/21 -> Degrees to Radians6/1  "<Latitude_GPS>"
  Bus Selector1/24 -> [FigureofMerit]  "<FigureofMerit>"
  [FigureofMerit] -> FigureofMerit/1
  Bus Selector1/25 -> RALTValid/1  "<RALTValid>"

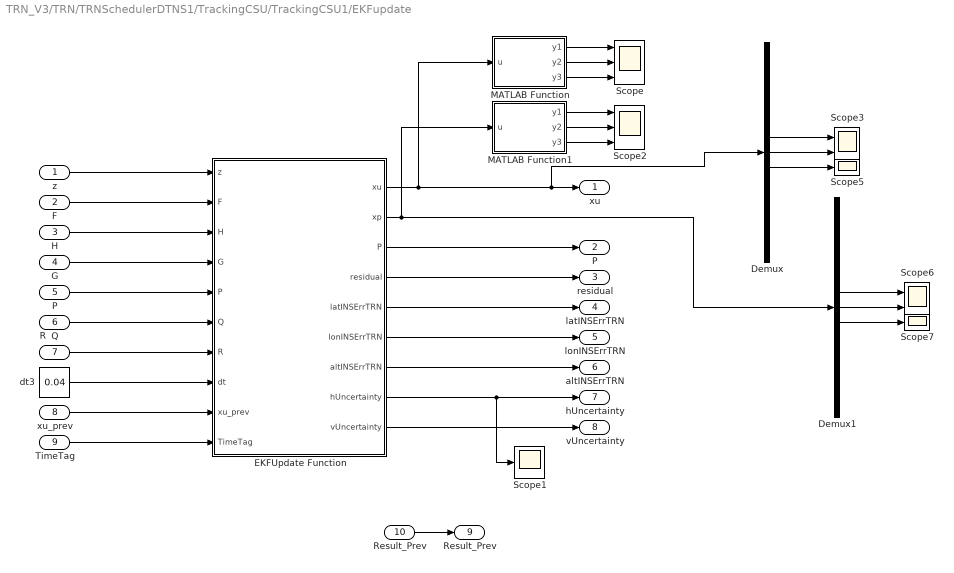
== system TRN_V3/TRN/TRNSchedulerDTNS1/TrackingCSU/TrackingCSU1/EKFupdate ==
  z : Inport
  F : Inport  Port=2
  H : Inport  Port=3
  G : Inport  Port=4
  "P " : Inport  Port=5
  Q : Inport  Port=6
  R : Inport  Port=7
  xu_prev : Inport  Port=8
  TimeTag : Inport  Port=9
  "Result_Prev " : Inport  Port=10
  Demux : Demux  Outputs=15
  Demux1 : Demux  Outputs=15
  EKFUpdate Function : MATLAB Function  TreatAsAtomicUnit=on
  MATLAB Function : MATLAB Function  TreatAsAtomicUnit=on
  MATLAB Function1 : MATLAB Function  TreatAsAtomicUnit=on
  Scope : Scope  NumInputPorts=3
  Scope1 : Scope
  Scope2 : Scope  NumInputPorts=3
  Scope3 : Scope  NumInputPorts=2
  Scope5 : Scope
  Scope6 : Scope  NumInputPorts=2
  Scope7 : Scope
  dt3 : Constant  Value=0.04  OutDataTypeStr=double
  xu : Outport
  P : Outport  Port=2
  residual : Outport  Port=3
  latINSErrTRN : Outport  Port=4
  lonINSErrTRN : Outport  Port=5
  altINSErrTRN : Outport  Port=6
  hUncertainty : Outport  Port=7
  vUncertainty : Outport  Port=8
  Result_Prev : Outport  Port=9
  wires:
  R/1 -> EKFUpdate Function/7(R)
  H/1 -> EKFUpdate Function/3(H)
  "P "/1 -> EKFUpdate Function/5("P ")
  EKFUpdate Function/9(vUncertainty) -> vUncertainty/1
  EKFUpdate Function/4(residual) -> residual/1
  TimeTag/1 -> EKFUpdate Function/10(TimeTag)
  F/1 -> EKFUpdate Function/2(F)
  xu_prev/1 -> EKFUpdate Function/9(xu_prev)
  G/1 -> EKFUpdate Function/4(G)
  EKFUpdate Function/1(xu) -> MATLAB Function/1(u), Demux/1, xu/1
  EKFUpdate Function/3(P) -> P/1
  Q/1 -> EKFUpdate Function/6(Q)
  z/1 -> EKFUpdate Function/1(z)
  dt3/1 -> EKFUpdate Function/8(dt)
  EKFUpdate Function/5(latINSErrTRN) -> latINSErrTRN/1
  EKFUpdate Function/6(lonINSErrTRN) -> lonINSErrTRN/1
  EKFUpdate Function/7(altINSErrTRN) -> altINSErrTRN/1
  EKFUpdate Function/8(hUncertainty) -> Scope1/1, hUncertainty/1
  "Result_Prev "/1 -> Result_Prev/1
  MATLAB Function/1(y1) -> Scope/1
  MATLAB Function/2(y2) -> Scope/2
  MATLAB Function/3(y3) -> Scope/3
  MATLAB Function1/1(y1) -> Scope2/1
  MATLAB Function1/2(y2) -> Scope2/2
  MATLAB Function1/3(y3) -> Scope2/3
  Demux/7 -> Scope3/1
  Demux/8 -> Scope3/2
  EKFUpdate Function/2(xp) -> MATLAB Function1/1(u), Demux1/1
  Demux/9 -> Scope5/1
  Demux1/9 -> Scope7/1
  Demux1/8 -> Scope6/2
  Demux1/7 -> Scope6/1

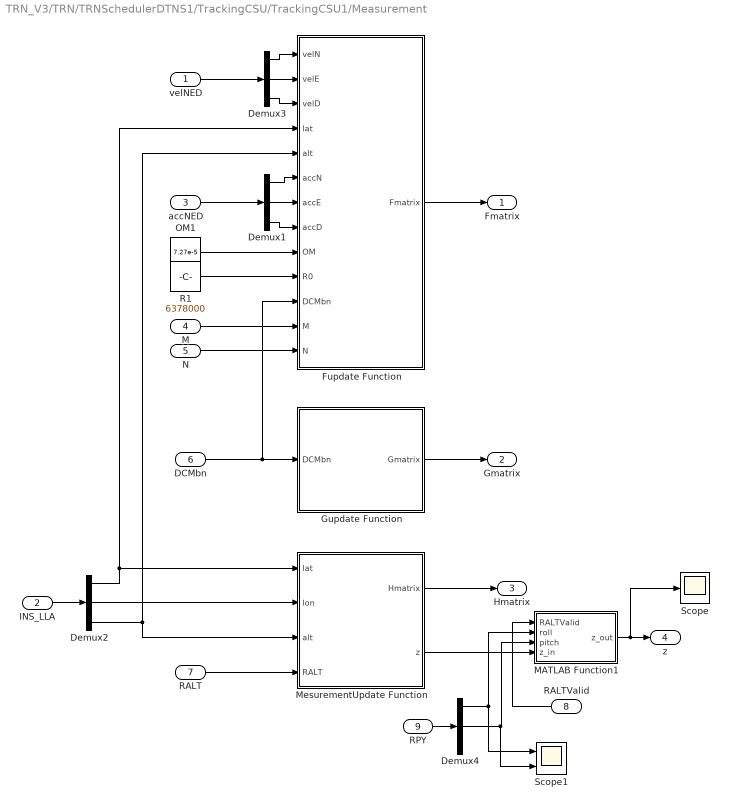
== system TRN_V3/TRN/TRNSchedulerDTNS1/TrackingCSU/TrackingCSU1/Measurement ==
  velNED : Inport
  INS_LLA : Inport  Port=2
  accNED : Inport  Port=3
  M : Inport  Port=4
  N : Inport  Port=5
  DCMbn : Inport  Port=6
  RALT : Inport  Port=7
  RALTValid : Inport  Port=8
  RPY : Inport  Port=9
  Demux{1..4} (4 alike) : Demux  Outputs=3
  Fupdate Function : MATLAB Function  TreatAsAtomicUnit=on
  Gupdate Function : MATLAB Function  TreatAsAtomicUnit=on
  MATLAB Function1 : MATLAB Function  TreatAsAtomicUnit=on
  MesurementUpdate Function : MATLAB Function  TreatAsAtomicUnit=on
  OM1 : Constant  Value=7.27e-5
  R1 : Constant  Value=6378000
  Scope : Scope
  Scope1 : Scope  NumInputPorts=2
  Fmatrix : Outport
  Gmatrix : Outport  Port=2
  Hmatrix : Outport  Port=3
  z : Outport  Port=4
  wires:
  Demux1/3 -> Fupdate Function/8(accD)
  OM1/1 -> Fupdate Function/9(OM)
  Demux3/1 -> Fupdate Function/1(velN)
  Demux1/2 -> Fupdate Function/7(accE)
  RALT/1 -> MesurementUpdate Function/4(RALT)
  Demux3/3 -> Fupdate Function/3(velD)
  Demux3/2 -> Fupdate Function/2(velE)
  Demux1/1 -> Fupdate Function/6(accN)
  Gupdate Function/1(Gmatrix) -> Gmatrix/1
  Fupdate Function/1(Fmatrix) -> Fmatrix/1
  DCMbn/1 -> Fupdate Function/11(DCMbn), Gupdate Function/1(DCMbn)
  N/1 -> Fupdate Function/13(N)
  accNED/1 -> Demux1/1
  velNED/1 -> Demux3/1
  M/1 -> Fupdate Function/12(M)
  MesurementUpdate Function/1(Hmatrix) -> Hmatrix/1
  R1/1 -> Fupdate Function/10(R0)
  RALTValid/1 -> MATLAB Function1/1(RALTValid)
  MesurementUpdate Function/2(z) -> MATLAB Function1/4(z_in)
  INS_LLA/1 -> Demux2/1
  Demux2/1 -> Fupdate Function/4(lat), MesurementUpdate Function/1(lat)
  Demux2/3 -> MesurementUpdate Function/3(alt), Fupdate Function/5(alt)
  Demux2/2 -> MesurementUpdate Function/2(lon)
  RPY/1 -> Demux4/1
  Demux4/1 -> MATLAB Function1/2(roll), Scope1/1
  Demux4/2 -> Scope1/2, MATLAB Function1/3(pitch)
  MATLAB Function1/1(z_out) -> z/1, Scope/1

== system TRN_V3/TRN/TRN_visualization /Subsystem1/If Action Subsystem ==
  LatErr : Inport
  LonErr : Inport  Port=2
  Action Port : ActionPort  ActionPortLabel=else
  Gain1 : Gain  Gain=3
  Gain2 : Gain  Gain=3
  Gain3 : Gain
  Gain4 : Gain  Gain=-1
  Gain6 : Gain
  Gain7 : Gain  Gain=-1
  Standard Deviation : dspstat3/Standard Deviation  run=on  directionMode=Entire input  dimension=1  reset_popup=None  roiEnable=off  roiType=Rectangles  roiPortion=Entire ROI  roiOutput=Individual statistics for each ROI  roiFlag=off
      settings: SourceProductBaseCode=DS
  Standard Deviation1 : dspstat3/Standard Deviation  run=on  directionMode=Entire input  dimension=1  reset_popup=None  roiEnable=off  roiType=Rectangles  roiPortion=Entire ROI  roiOutput=Individual statistics for each ROI  roiFlag=off
      settings: SourceProductBaseCode=DS
  Out1 : Outport
  Out3 : Outport  Port=2
  Out5 : Outport  Port=3
  Out7 : Outport  Port=4
  wires:
  LatErr/1 -> Standard Deviation/1
  LonErr/1 -> Standard Deviation1/1
  Gain6/1 -> Out5/1
  Gain2/1 -> Gain4/1, Gain3/1
  Gain7/1 -> Out7/1
  Standard Deviation1/1 -> Gain1/1
  Standard Deviation/1 -> Gain2/1
  Gain3/1 -> Out1/1
  Gain4/1 -> Out3/1
  Gain1/1 -> Gain7/1, Gain6/1

== system TRN_V3/TRN/TRN_visualization /Subsystem1/If Action Subsystem1 ==
  Action Port : ActionPort  ActionPortLabel=if(u1 > 0)
  Constant : Constant  Value=0
  Out1 : Outport
  Out2 : Outport  Port=2
  Out3 : Outport  Port=3
  Out4 : Outport  Port=4
  wires:
  Constant/1 -> Out4/1, Out3/1, Out2/1, Out1/1

== system TRN_V3/TRN/TRN_visualization /Subsystem1/If Action Subsystem2 ==
  LatErr : Inport
  LonErr : Inport  Port=2
  Action Port : ActionPort  ActionPortLabel=else
  Out1 : Outport
  Out5 : Outport  Port=2
  wires:
  LonErr/1 -> Out5/1
  LatErr/1 -> Out1/1

== system TRN_V3/TRN/TRN_visualization /Subsystem1/If Action Subsystem3 ==
  Action Port : ActionPort  ActionPortLabel=if(u1 < 0)
  Constant : Constant  Value=0
  Out1 : Outport
  Out2 : Outport  Port=2
  wires:
  Constant/1 -> Out2/1, Out1/1

== matlab function TRN_V3/DataProcess/Subsystem3/Flag_WoW ==
  data: time input; WeightOnWheels output
function WeightOnWheels  = fcn(time)

% WeightOnWheels
% False[0]_flight / True[1]_ground

if time <= 30
    WeightOnWheels = boolean(true);
else
    WeightOnWheels = boolean(false);
end

end

== matlab function TRN_V3/TRN/INS//GPSFilter/MATLAB Function2 ==
  data: FoM input; out_GPSpos output; EstHorErr input; EstVerErr input; state input; in_GPSpos input; in_GPSvel input; out_GPSvel output; GPSDataNotValid input
function [out_GPSpos, out_GPSvel] = GPScheck(FoM, EstHorErr, EstVerErr, state, in_GPSpos, in_GPSvel, GPSDataNotValid)

if GPSDataNotValid == 0
    if EstHorErr < 100 && EstVerErr < 25 && state == 5
        if FoM < 4
            out_GPSpos = in_GPSpos;
            out_GPSvel = zeros(3,1);
            if FoM < 2
                out_GPSpos = in_GPSpos;
                out_GPSvel = in_GPSvel;
            end
        else
            out_GPSpos = zeros(3,1);
            out_GPSvel = zeros(3,1);
        end
    else
        out_GPSpos = zeros(3,1);
        out_GPSvel = zeros(3,1);
    end
else
    out_GPSpos = zeros(3,1);
    out_GPSvel = zeros(3,1);
end

== matlab function TRN_V3/DataProcess/Subsystem3/MATLAB Function ==
  data: count input; count output
function count = fcn(count)

count = count + 0.04;

== matlab function TRN_V3/DataProcess/Subsystem3/Subsystem1/MATLAB Function3 ==
  data: u input; a output; b output
function [a,b]  = fcn(u)

% WeightOnWheels
if(u==1)
    a = boolean(true);
    b = boolean(true);
else
    a = boolean(false);
    b = boolean(false);
end

end

== matlab function TRN_V3/DataProcess/Subsystem3/Subsystem1/MATLAB Function1 ==
  data: WoW input; time input; lat_bias output; lon_bias output
function [lat_bias,lon_bias] = fcn(WoW, time)
%% parameters
lat2m = 111000;
lon2m = 91170;
bias1 = 500;   % 500m
bias2 = 500;   % 500m

%%
if time > 60
    if WoW == 0                % 0_flight / 1_ground
        lat_bias = bias1/lat2m;
        lon_bias = bias2/lon2m;
    else
        lat_bias = 0;
        lon_bias = 0;
    end
else
    lat_bias = 0;
    lon_bias = 0;
end

== matlab function TRN_V3/TRN/MATLAB Function ==
  data: u input; yy output
function yy = fcn(u)
    y = diag(u);
    yy = [y(7), y(8), y(9)./(6378000)];

    yy = yy.*(6378000*25);

end

== matlab function TRN_V3/TRN/MATLAB Function1 ==
  data: latINS input; TRNEstOfLatErr output; lonINS input; altINS input; latGPS input; lonGPS input; altGPS input; flagGPS input; TRNEstOfLonErr output; TRNEstOfaltErr output; roll input; pitch input
function [TRNEstOfLatErr, TRNEstOfLonErr, TRNEstOfaltErr] = fcn(latINS, lonINS, altINS,  latGPS, lonGPS, altGPS, flagGPS, roll, pitch)

if abs(roll) < 15 && abs(pitch) < 15
    TRNEstOfLatErr = latINS;
    TRNEstOfLonErr = lonINS;
    TRNEstOfaltErr = altINS;
    if flagGPS ==0
      TRNEstOfLatErr = latGPS;
      TRNEstOfLonErr = lonGPS;
      TRNEstOfaltErr = altGPS;
    end
else
    TRNEstOfLatErr = 0;
    TRNEstOfLonErr = 0;
    TRNEstOfaltErr = 0;
end

== matlab function TRN_V3/TRN/MATLAB Function2 ==
  data: INS_Mech_flag input; TRN_valid output; Latitude_INS input
function TRN_valid = fcn(INS_Mech_flag, Latitude_INS)

    if( abs(Latitude_INS) > 80.0)
        Latitude_INS_flag = 0;
    else
        Latitude_INS_flag = 1;
    end

    if( (INS_Mech_flag < 1) || (Latitude_INS_flag < 1))
        TRN_valid = boolean(false);
    else
        TRN_valid = boolean(true);
    end

end

== matlab function TRN_V3/TRN/INS//GPSFilter/EKFUpdate Function ==
  data: xu input; xu output; z input; P_out output; F input; H input; G input; P input; Q input; R input; dt input; LCI_lat output; LCI_lon output; LCI_alt output
% function [xu, P, residual, LCI_lat, LCI_lon, LCI_alt] = EKFUpdate(z, F, H, G, P, Q, R, dt, xu_prev, TimeTag)
function [xu, P_out, LCI_lat, LCI_lon, LCI_alt] = EKFUpdate(xu, z, F, H, G, P, Q, R, dt)

x = xu;
I = eye(max(size(F)));

A = I + (F*dt);
Qk = (A*G * Q * G'*A') .* dt;

%-------------------------------------%
% Predicts states & covariance matrix
%-------------------------------------%
xp = A * x;
Pp = (A * P * A') + Qk;

%---------------------%
% Updates Kalman gain
%---------------------%
K = (Pp * H')/(R + H * Pp * H');

%----------------%
% Updates states
%----------------%
xu = xp + K * (z - H*xp);
% residual = z;

%---------------------------%
% Updates covariance matrix
%---------------------------%
% P_out = (I - K*H) * Pp * (I - K*H)' + K*R*K';
P_out = (I - K*H)*Pp;


LCI_lat = xu(1);
LCI_lon = xu(2);
LCI_alt = xu(3);
    
% if TimeTag(6) == 1
%     xu = xu_prev;
%     latINSErrTRN = xu(7);
%     lonINSErrTRN = xu(8);
%     altINSErrTRN = xu(9);
% end

end

== matlab function TRN_V3/TRN/MATLAB Function4 ==
  data: P input; hUncertainty output; vUncertainty output
function [hUncertainty,vUncertainty] = fcn(P)

hUncertainty = sqrt(abs(P(7,7) + P(8,8))) * 6378000;
vUncertainty = sqrt(abs(P(9,9)));

== matlab function TRN_V3/TRN/INSValidCheck/MATLAB Function5 ==
  data: diff_Lat input; NotValid output; diff_Lon input; Valid input; in_count input; out_count output
function [NotValid,out_count] = INSValidCheck(diff_Lat,diff_Lon,Valid,in_count)
out_count = 0;
NotValid = boolean(false);
lat2m = 111000;
lon2m = 91170;

if Valid == 0                       % INS Notvalid [5sec]
    NotValid = boolean(false);      % Init Setting
    out_count = in_count + 1;
    if out_count > (5*25)
        NotValid = boolean(true);   % INS Notvalid
    end
elseif (abs(diff_Lat*lat2m) > 100 || abs(diff_Lon*lon2m) > 100)                  % INS Switch
    NotValid = boolean(true);
elseif Valid > 0 && (abs(diff_Lat*lat2m) <= 100 && abs(diff_Lon*lon2m) <= 100)   % INS valid
    NotValid = boolean(false);                                                   % INS valid
end

== matlab function TRN_V3/TRN/Subsystem/FTGMapCaching ==
  data: resultDTED output; resultDVOF output; lat input; lon input; hDEM output
function [resultDTED, resultDVOF, hDEM] = FTGMapCaching(lat, lon)

resultDTED = uint32(1);
resultDVOF = int32(1);
hDEM = double(0.0);                                 %%20220419

resultDVOF = coder.ceval('UpdateObstList', lat, lon);
resultDTED = coder.ceval('UpdateMapCache', lat, lon);
hDEM = coder.ceval('GetElevation', lat, lon);       %%20220419

== matlab function TRN_V3/TRN/Subsystem/MATLAB Function ==
  data: Resolution output; Map_Size output; bottomLat output; leftLon output
function [Resolution, Map_Size, bottomLat, leftLon] = ReturnBottomLeftLatLon

Resolution = double(0.0);
Map_Size = double(0.0);

leftLon = 0.0;
leftLon = coder.ceval('ReturnLeftLon');

bottomLat = 0.0;
bottomLat = coder.ceval('ReturnBottomLat');

end

== matlab function TRN_V3/TRN/TRN_visualization /MATLAB Function ==
  data: Err_Lat_INS output; Err_Lon_INS output; Err_Alt_INS output; lat_Ref input; lon_Ref input; alt_Ref input; lat_INS input; lon_INS input; alt_INS input; Lat_INS output; Lon_INS output; Alt_INS output; Lat_Ref output; Lon_Ref output; Alt_Ref output
function [Err_Lat_INS, Err_Lon_INS, Err_Alt_INS, Lat_INS, Lon_INS, Alt_INS, Lat_Ref, Lon_Ref, Alt_Ref] = fcn(lat_Ref, lon_Ref, alt_Ref, lat_INS, lon_INS, alt_INS)

%% parameters
lat2m = 111000;
lon2m = 91170;

%% 초기값 setting
% init_lat = 35.1;
% init_lon = 128.5;
% init_alt = 1000;

Lat_INS = lat_INS;               % INS Latitude
Lon_INS = lon_INS;               % INS Longitude
% Alt_INS = uint16(alt_INS);               % INS Altitude
Alt_INS = alt_INS;               % INS Altitude

Lat_Ref = lat_Ref;             % Ref Latitude
Lon_Ref = lon_Ref;             % Ref Longitude
% Alt_Ref = uint16(alt_Ref);             % Ref Altitude
Alt_Ref = alt_Ref;             % Ref Altitude

Err_Lat_INS = (Lat_Ref-Lat_INS)*lat2m;
Err_Lon_INS = (Lon_Ref-Lon_INS)*lon2m;
Err_Alt_INS = (Alt_Ref-Alt_INS);

end

== matlab function TRN_V3/TRN/TRN_visualization /MATLAB Function1 ==
  data: x input; a output; y input
function a = fcn(x,y)

a = sqrt(x^2+y^2);

== matlab function TRN_V3/TRN/TRN_visualization /MATLAB Function2 ==
  data: x input; a output; y input
function a = fcn(x,y)

a = sqrt(x^2+y^2);

== matlab function TRN_V3/TRN/TRN_visualization /Terrain_Level_big4 ==
  data: Lat input; Lon input; R output
function R = Terrain_level_big1(Lat, Lon)

    R = Terrain_level(Lat, Lon);

end
